simulink model "gm_sampleModel1671_3_sub"  (R2023a)
settings: Solver=VariableStepAuto  StartTime=0.0  StopTime=10.0  RelTol=1e-3
libraries: simulink x1, hdlsllib x1
settings Model: Creator=user1  LastModifiedBy=user1
settings OptimizationCC: BlockReduction=off  ConditionallyExecuteInputs=off
settings DebuggingCC: InheritedTsInSrcMsg=none

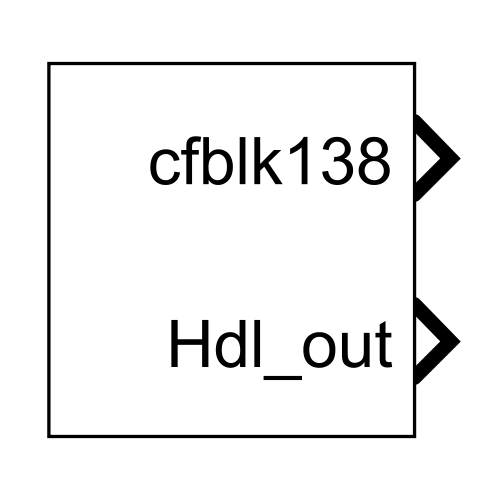
[thumbnail: Simulink's stored preview of the top-level diagram]
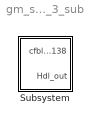
== system gm_sampleModel1671_3_sub ==
  Subsystem : Subsystem

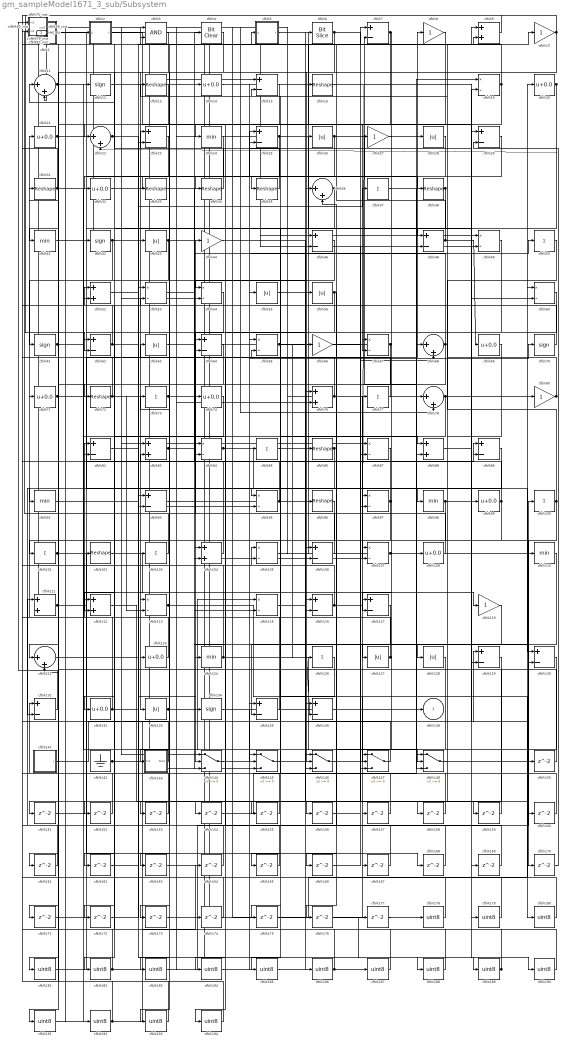
== system gm_sampleModel1671_3_sub/Subsystem ==
  cfblk1 : Subsystem  mask(Detect Fall Negative){vinit=double(0), InputProcessing=Elements as channels (sample based), OutDataTypeStr=uint8}
      mask prompts: vinit "Simulink:masks:InitialCondition_MP"; InputProcessing "Simulink:masks:InputProcessing_MP"; OutDataTypeStr "Simulink:masks:OutputDataType_MP"
      mask help: Simulink:masks:DetectFallNegative_MD
      mask init:
      | InputProcessing = 'Elements as channels (sample based)';
      | OutDataTypeStr = 'uint8';
      | vinit = double(0);
      mask TypeOptions InputProcessing: Simulink:masks:ColumnsAsChannelsFrameBased | Simulink:masks:ElementsAsChannelsSampleBased
      mask TypeOptions OutDataTypeStr: Simulink:masks:uint8 | Simulink:masks:boolean
      mask Display: fprintf('U < 0\n&  NOT\nU/z < 0')
  cfblk{8,10,27,44,66,80,119} (7 alike) : Gain  OutDataTypeStr=uint8
  cfblk{37,50,73,77,85,100..101,103,126} (9 alike) : Sum  Inputs=+  OutDataTypeStr=uint8
  cfblk{13,16,31,33..35,38,72,86,96,102} (11 alike) : Reshape
  cfblk{9,52,76,83,88,104,111..112} (8 alike) : Sum  OutDataTypeStr=uint8
  cfblk{19,49,53..54,60,65,67,84,87,95,97,105,107,113,115} (15 alike) : Product  Inputs=*/  OutDataTypeStr=uint8  RndMeth=Zero  SaturateOnIntegerOverflow=on
  cfblk{7,15,23,25,29,46,48,62,64,82,89,93,106,116..117,129..131,135..136} (20 alike) : Sum  Inputs=+-  OutDataTypeStr=uint8
  cfblk{14,20..21,32,69,71,74,99,108,123,132} (11 alike) : Bias  Bias=0.0  SaturateOnIntegerOverflow=off
  cfblk{11,22,36,68,78,121} (6 alike) : Sum  Inputs=|++  OutDataTypeStr=uint8
  cfblk{24,41,91,98,110,124} (6 alike) : MinMax  OutDataTypeStr=uint8
  cfblk114_inst : Subsystem
  cfblk118_inst : Subsystem
  cfblk{12,42,61,70,134} (5 alike) : Signum
  cfblk122_inst : Subsystem
  cfblk125_inst : Subsystem
  cfblk{26,28,43,55..56,63,127..128,133} (9 alike) : Abs  OutDataTypeStr=uint8  SaturateOnIntegerOverflow=off
  cfblk141 : Subsystem  mask(Counter Limited){uplimit=double(7), tsamp=double(-1)}
      mask prompts: uplimit "Simulink:masks:UpperLimit_MP"; tsamp "Simulink:masks:SampleTime_MP"
      mask help: Simulink:masks:CounterLimited_MD
      mask init:
      | nbits = double(8);
      | tsamp = double(-1);
      | uplimit = double(7);
  cfblk142 : Ground
  cfblk143 : Subsystem
  cfblk{144..148} (5 alike) : Switch  OutDataTypeStr=uint8  SaturateOnIntegerOverflow=off  InputSameDT=off
  cfblk{150..177} (28 alike) : Delay  SampleTime=1
  cfblk{178..194} (17 alike) : DataTypeConversion  OutDataTypeStr=uint8  SaturateOnIntegerOverflow=off  RndMeth=Floor
  cfblk17_inst : Subsystem
  cfblk18_inst : Subsystem
  cfblk2 : Subsystem  mask(Detect Fall Nonpositive){vinit=double(0), InputProcessing=Elements as channels (sample based), OutDataTypeStr=uint8}
      mask prompts: vinit "Simulink:masks:InitialCondition_MP"; InputProcessing "Simulink:masks:InputProcessing_MP"; OutDataTypeStr "Simulink:masks:OutputDataType_MP"
      mask help: Simulink:masks:DetectFallNonpositive_MD
      mask init:
      | InputProcessing = 'Elements as channels (sample based)';
      | OutDataTypeStr = 'uint8';
      | vinit = double(0);
      mask TypeOptions InputProcessing: Simulink:masks:ColumnsAsChannelsFrameBased | Simulink:masks:ElementsAsChannelsSampleBased
      mask TypeOptions OutDataTypeStr: Simulink:masks:uint8 | Simulink:masks:boolean
      mask Display: fprintf('U <= 0\n&  NOT\nU/z <= 0')
  cfblk3 : Logic  AllPortsSameDT=off  OutDataTypeStr=boolean
  cfblk30_inst : Subsystem
  cfblk39_inst : Subsystem
  cfblk4 : simulink/Logic and Bit Operations/Bit Clear  iBit=0
      settings: LibrarySourceBlock=|
      | hdlsllib/Logic and Bit
      | Operations/Bit Clear
  cfblk40_inst : Subsystem
  cfblk45_inst : Subsystem
  cfblk47_inst : Subsystem
  cfblk5 : Subsystem  mask(Detect Fall Negative){vinit=double(0), InputProcessing=Elements as channels (sample based), OutDataTypeStr=uint8}
      mask prompts: vinit "Simulink:masks:InitialCondition_MP"; InputProcessing "Simulink:masks:InputProcessing_MP"; OutDataTypeStr "Simulink:masks:OutputDataType_MP"
      mask help: Simulink:masks:DetectFallNegative_MD
      mask init:
      | InputProcessing = 'Elements as channels (sample based)';
      | OutDataTypeStr = 'uint8';
      | vinit = double(0);
      mask TypeOptions InputProcessing: Simulink:masks:ColumnsAsChannelsFrameBased | Simulink:masks:ElementsAsChannelsSampleBased
      mask TypeOptions OutDataTypeStr: Simulink:masks:uint8 | Simulink:masks:boolean
      mask Display: fprintf('U < 0\n&  NOT\nU/z < 0')
  cfblk51_inst : Subsystem
  cfblk57_inst : Subsystem
  cfblk59_inst : Subsystem
  cfblk6 : hdlsllib/Logic and Bit Operations/Bit Slice  lidx=7  ridx=0
  cfblk75_inst : Subsystem
  cfblk79_inst : Subsystem
  cfblk90_inst : Subsystem
  cfblk92_inst : Subsystem
  cfblk138 : Outport  OutDataTypeStr=uint8  SampleTime=1  VectorParamsAs1DForOutWhenUnconnected=off
  Hdl_out : Outport  Port=2  OutDataTypeStr=uint8  SampleTime=1
  wires:
  cfblk1/1(Y) -> cfblk88/1, cfblk95/1
  cfblk10/1 -> cfblk62/2, cfblk146/2, cfblk133/1
  cfblk100/1 -> cfblk123/1, cfblk53/2, cfblk170/1
  cfblk101/1 -> cfblk8/1, cfblk168/1
  cfblk102/1 -> cfblk116/1
  cfblk103/1 -> cfblk59_inst/2(in2)
  cfblk104/1 -> cfblk83/2
  cfblk105/1 -> cfblk10/1
  cfblk106/1 -> cfblk44/1
  cfblk107/1 -> cfblk108/1, cfblk19/1
  cfblk108/1 -> cfblk23/1
  cfblk11/1 -> cfblk76/1, cfblk144/2
  cfblk110/1 -> cfblk135/2
  cfblk111/1 -> cfblk12/1, cfblk65/2
  cfblk112/1 -> cfblk154/1
  cfblk113/1 -> cfblk55/1, cfblk180/1
  cfblk114_inst/1(out1) -> cfblk186/1
  cfblk115/1 -> cfblk106/2
  cfblk116/1 -> cfblk7/2, cfblk45_inst/2(in2)
  cfblk117/1 -> cfblk185/1
  cfblk118_inst/1(out1) -> cfblk192/1
  cfblk119/1 -> cfblk128/1
  cfblk12/1 -> cfblk24/1
  cfblk121/1 -> cfblk146/1
  cfblk122_inst/1(out1) -> cfblk84/1
  cfblk123/1 -> cfblk21/1
  cfblk124/1 -> cfblk71/1, cfblk148/2, cfblk136/2, cfblk177/1
  cfblk125_inst/1(out1) -> cfblk74/1, cfblk111/2, cfblk11/2
  cfblk126/1 -> cfblk165/1
  cfblk127/1 -> cfblk82/1, cfblk15/2
  cfblk128/1 -> cfblk166/1
  cfblk129/1 -> cfblk151/1
  cfblk13/1 -> cfblk41/1
  cfblk130/1 -> cfblk167/1
  cfblk131/1 -> cfblk79_inst/1(in1)
  cfblk132/1 -> cfblk40_inst/2(in2), cfblk159/1
  cfblk133/1 -> cfblk146/3, cfblk115/1
  cfblk134/1 -> cfblk145/1
  cfblk135/1 -> cfblk57_inst/1(in1)
  cfblk136/1 -> cfblk78/1
  cfblk14/1 -> cfblk38/1
  cfblk141/1(y) -> cfblk116/2
  cfblk142/1 -> cfblk129/1, cfblk19/2
  cfblk143/1(Out1) -> cfblk125_inst/1(in1)
  cfblk144/1 -> cfblk70/1
  cfblk145/1 -> cfblk157/1
  cfblk146/1 -> cfblk77/1
  cfblk147/1 -> cfblk136/1
  cfblk148/1 -> cfblk100/1
  cfblk15/1 -> cfblk54/1
  cfblk150/1 -> cfblk122_inst/2(in2)
  cfblk151/1 -> cfblk25/2
  cfblk152/1 -> cfblk131/1
  cfblk153/1 -> cfblk79_inst/2(in2)
  cfblk154/1 -> cfblk88/2
  cfblk155/1 -> cfblk84/2
  cfblk156/1 -> cfblk68/1
  cfblk157/1 -> cfblk57_inst/2(in2)
  cfblk158/1 -> cfblk51_inst/1(in1)
  cfblk159/1 -> cfblk75_inst/1(in1)
  cfblk16/1 -> cfblk190/1
  cfblk160/1 -> cfblk105/1
  cfblk161/1 -> cfblk40_inst/1(in1)
  cfblk162/1 -> cfblk93/1
  cfblk163/1 -> cfblk135/1
  cfblk164/1 -> cfblk3/1
  cfblk165/1 -> cfblk92_inst/2(in2)
  cfblk166/1 -> cfblk48/2
  cfblk167/1 -> cfblk64/1
  cfblk168/1 -> cfblk111/1
  cfblk169/1 -> cfblk36/2
  cfblk17_inst/1(out1) -> cfblk43/1, cfblk138/1
  cfblk170/1 -> cfblk29/2
  cfblk171/1 -> cfblk23/2
  cfblk172/1 -> cfblk83/1
  cfblk173/1 -> cfblk46/2
  cfblk174/1 -> cfblk62/1
  cfblk175/1 -> cfblk60/1
  cfblk176/1 -> cfblk188/1
  cfblk177/1 -> cfblk1/1(U)
  cfblk178/1 -> cfblk53/1
  cfblk179/1 -> cfblk18_inst/1(in1)
  cfblk18_inst/1(out1) -> cfblk178/1
  cfblk180/1 -> cfblk18_inst/2(in2)
  cfblk181/1 -> cfblk4/1
  cfblk182/1 -> cfblk17_inst/2(in2), cfblk105/2
  cfblk183/1 -> cfblk150/1
  cfblk184/1 -> cfblk89/1
  cfblk185/1 -> cfblk89/2
  cfblk186/1 -> cfblk39_inst/2(in2), cfblk122_inst/1(in1)
  cfblk187/1 -> cfblk114_inst/1(in1)
  cfblk188/1 -> cfblk114_inst/2(in2)
  cfblk189/1 -> cfblk90_inst/2(in2), cfblk164/1
  cfblk19/1 -> cfblk45_inst/1(in1), cfblk147/2
  cfblk190/1 -> cfblk52/1
  cfblk191/1 -> cfblk52/2
  cfblk192/1 -> cfblk31/1, cfblk20/1, cfblk174/1
  cfblk193/1 -> cfblk118_inst/1(in1)
  cfblk194/1 -> cfblk118_inst/2(in2)
  cfblk2/1(Y) -> cfblk179/1
  cfblk20/1 -> cfblk22/2, cfblk144/3, cfblk175/1
  cfblk21/1 -> cfblk48/1, cfblk34/1
  cfblk22/1 -> cfblk147/3, cfblk134/1
  cfblk23/1 -> cfblk72/1
  cfblk24/1 -> cfblk193/1
  cfblk25/1 -> cfblk99/1, cfblk93/2
  cfblk26/1 -> cfblk9/2, cfblk148/1, cfblk173/1, cfblk172/1
  cfblk27/1 -> cfblk107/1
  cfblk28/1 -> cfblk36/1
  cfblk29/1 -> cfblk32/1
  cfblk3/1 -> cfblk191/1
  cfblk30_inst/1(out1) -> cfblk42/1
  cfblk31/1 -> cfblk39_inst/1(in1), cfblk171/1, cfblk113/1
  cfblk32/1 -> cfblk35/1
  cfblk33/1 -> cfblk56/1
  cfblk34/1 -> cfblk11/1
  cfblk35/1 -> cfblk51_inst/2(in2)
  cfblk36/1 -> cfblk194/1, cfblk124/1
  cfblk37/1 -> cfblk129/2
  cfblk38/1 -> cfblk112/2, cfblk153/1
  cfblk39_inst/1(out1) -> cfblk26/1, cfblk144/1
  cfblk4/1 -> cfblk182/1
  cfblk40_inst/1(out1) -> cfblk76/2, cfblk54/2
  cfblk41/1 -> cfblk102/1
  cfblk42/1 -> cfblk121/2, cfblk5/1(U)
  cfblk43/1 -> cfblk7/1, cfblk61/1
  cfblk44/1 -> cfblk147/1
  cfblk45_inst/1(out1) -> cfblk14/1
  cfblk46/1 -> cfblk132/1
  cfblk47_inst/1(out1) -> cfblk95/2, cfblk2/1(U)
  cfblk48/1 -> cfblk69/1, cfblk47_inst/1(in1)
  cfblk49/1 -> cfblk97/1
  cfblk5/1(Y) -> cfblk67/2
  cfblk50/1 -> cfblk158/1
  cfblk51_inst/1(out1) -> cfblk187/1, cfblk27/1
  cfblk52/1 -> cfblk189/1
  cfblk53/1 -> cfblk97/2
  cfblk54/1 -> cfblk64/2
  cfblk55/1 -> cfblk6/1
  cfblk56/1 -> cfblk104/1, cfblk176/1
  cfblk57_inst/1(out1) -> cfblk28/1, cfblk87/1
  cfblk59_inst/1(out1) -> cfblk30_inst/1(in1), cfblk145/3
  cfblk6/1 -> cfblk148/3, cfblk163/1
  cfblk60/1 -> cfblk66/1
  cfblk61/1 -> cfblk117/2, cfblk161/1
  cfblk62/1 -> cfblk33/1, cfblk30_inst/2(in2)
  cfblk63/1 -> cfblk50/1
  cfblk64/1 -> cfblk143/1(In1)
  cfblk65/1 -> cfblk130/2, cfblk119/1, cfblk126/1
  cfblk66/1 -> cfblk68/2
  cfblk67/1 -> cfblk121/1, cfblk117/1, Hdl_out/1
  cfblk68/1 -> cfblk25/1, cfblk112/1
  cfblk69/1 -> cfblk98/1
  cfblk7/1 -> cfblk67/1, cfblk103/1
  cfblk70/1 -> cfblk90_inst/1(in1)
  cfblk71/1 -> cfblk145/2, cfblk87/2
  cfblk72/1 -> cfblk92_inst/1(in1), cfblk113/2
  cfblk73/1 -> cfblk9/1, cfblk3/2, cfblk115/2
  cfblk74/1 -> cfblk162/1
  cfblk75_inst/1(out1) -> cfblk80/1, cfblk49/1, cfblk107/2
  cfblk76/1 -> cfblk17_inst/1(in1), cfblk160/1
  cfblk77/1 -> cfblk63/1
  cfblk78/1 -> cfblk156/1, cfblk155/1
  cfblk79_inst/1(out1) -> cfblk75_inst/2(in2), cfblk16/1, cfblk49/2
  cfblk8/1 -> cfblk22/1
  cfblk80/1 -> cfblk47_inst/2(in2), cfblk13/1
  cfblk82/1 -> cfblk65/1
  cfblk83/1 -> cfblk46/1, cfblk127/1
  cfblk84/1 -> cfblk130/1, cfblk85/1
  cfblk85/1 -> cfblk86/1
  cfblk86/1 -> cfblk184/1, cfblk131/2
  cfblk87/1 -> cfblk181/1
  cfblk88/1 -> cfblk60/2
  cfblk89/1 -> cfblk183/1
  cfblk9/1 -> cfblk59_inst/1(in1)
  cfblk90_inst/1(out1) -> cfblk96/1
  cfblk91/1 -> cfblk37/1
  cfblk92_inst/1(out1) -> cfblk78/2, cfblk15/1, cfblk110/1
  cfblk93/1 -> cfblk29/1
  cfblk95/1 -> cfblk82/2, cfblk73/1
  cfblk96/1 -> cfblk106/1
  cfblk97/1 -> cfblk152/1, cfblk91/1
  cfblk98/1 -> cfblk169/1, cfblk101/1
  cfblk99/1 -> cfblk125_inst/2(in2), cfblk104/2

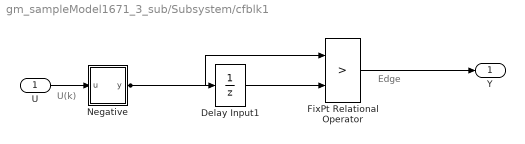
== system gm_sampleModel1671_3_sub/Subsystem/cfblk1 ==
  note: U(k)
  note: Edge
  U : Inport  OutDataTypeStr=uint8  SampleTime=1
  Delay Input1 : UnitDelay  Description=Store in Global RAM  DisableCoverage=on  InitialCondition=vinit  SampleTime=-1  HasFrameUpgradeWarning=on
  FixPt Relational Operator : RelationalOperator  Operator=>  OutDataTypeStr=fixdt(0, 8)  ZeroCross=off  InputSameDT=off
  Negative : Subsystem  mask(Compare To Zero){relop=<, OutDataTypeStr=boolean, ZeroCross=off}
      mask prompts: relop "Simulink:masks:Operator_MP"; OutDataTypeStr "Simulink:masks:OutputDataType_MP"; ZeroCross "Simulink:masks:EnableZerocrossingDetection_MP"
      mask help: Simulink:masks:CompareToZero_MD
      mask init:
      | OutDataTypeStr = 'boolean';
      | ZeroCross = 'off';
      | blkName = 'sampleModel1671_3_sub/Subsystem/cfblk1/Negative';
      | relop = '<';
      | setValue = 'boolean';
      mask TypeOptions relop: == | ~= | < | <= | >= | >
      mask TypeOptions OutDataTypeStr: Simulink:masks:uint8 | Simulink:masks:boolean
      mask Callback ZeroCross: sl('zeroCrossEnable', gcbh);
      mask Display: disp([relop,' 0'])
  Y : Outport  SampleTime=1
  wires:
  U/1 -> Negative/1(u)
  Delay Input1/1 -> FixPt Relational Operator/2
  FixPt Relational Operator/1 -> Y/1
  Negative/1(y) -> FixPt Relational Operator/1, Delay Input1/1

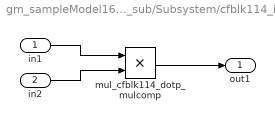
== system gm_sampleModel1671_3_sub/Subsystem/cfblk114_inst ==
  in1 : Inport  OutDataTypeStr=uint8  SampleTime=1
  in2 : Inport  Port=2  OutDataTypeStr=uint8  SampleTime=1
  mul_cfblk114_dotp_mulcomp : Product  Inputs=**  OutDataTypeStr=uint8  SampleTime=1
  out1 : Outport  OutDataTypeStr=uint8  SampleTime=1
  wires:
  in1/1 -> mul_cfblk114_dotp_mulcomp/1
  in2/1 -> mul_cfblk114_dotp_mulcomp/2
  mul_cfblk114_dotp_mulcomp/1 -> out1/1

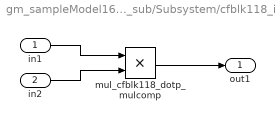
== system gm_sampleModel1671_3_sub/Subsystem/cfblk118_inst ==
  in1 : Inport  OutDataTypeStr=uint8  SampleTime=1
  in2 : Inport  Port=2  OutDataTypeStr=uint8  SampleTime=1
  mul_cfblk118_dotp_mulcomp : Product  Inputs=**  OutDataTypeStr=uint8  SampleTime=1
  out1 : Outport  OutDataTypeStr=uint8  SampleTime=1
  wires:
  in1/1 -> mul_cfblk118_dotp_mulcomp/1
  in2/1 -> mul_cfblk118_dotp_mulcomp/2
  mul_cfblk118_dotp_mulcomp/1 -> out1/1

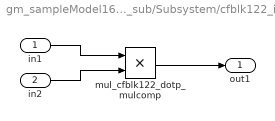
== system gm_sampleModel1671_3_sub/Subsystem/cfblk122_inst ==
  in1 : Inport  OutDataTypeStr=uint8  SampleTime=1
  in2 : Inport  Port=2  OutDataTypeStr=uint8  SampleTime=1
  mul_cfblk122_dotp_mulcomp : Product  Inputs=**  OutDataTypeStr=uint8  SampleTime=1
  out1 : Outport  OutDataTypeStr=uint8  SampleTime=1
  wires:
  in1/1 -> mul_cfblk122_dotp_mulcomp/1
  in2/1 -> mul_cfblk122_dotp_mulcomp/2
  mul_cfblk122_dotp_mulcomp/1 -> out1/1

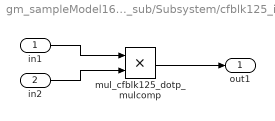
== system gm_sampleModel1671_3_sub/Subsystem/cfblk125_inst ==
  in1 : Inport  OutDataTypeStr=uint8  SampleTime=1
  in2 : Inport  Port=2  OutDataTypeStr=uint8  SampleTime=1
  mul_cfblk125_dotp_mulcomp : Product  Inputs=**  OutDataTypeStr=uint8  SampleTime=1
  out1 : Outport  OutDataTypeStr=uint8  SampleTime=1
  wires:
  in1/1 -> mul_cfblk125_dotp_mulcomp/1
  in2/1 -> mul_cfblk125_dotp_mulcomp/2
  mul_cfblk125_dotp_mulcomp/1 -> out1/1

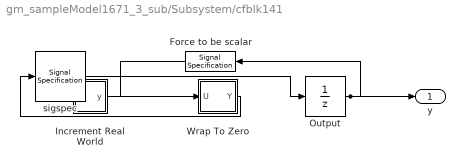
== system gm_sampleModel1671_3_sub/Subsystem/cfblk141 ==
  Force to be scalar : SignalSpecification  DisableCoverage=on  Dimensions=1
  Increment Real World : Subsystem  mask(Real World Value Increment){}
      mask help: Simulink:masks:RealWorldValueIncrement_MD
      mask Display: disp('V++')
  Output : UnitDelay  InitialCondition=0.0  SampleTime=tsamp  HasFrameUpgradeWarning=on
  Wrap To Zero : Subsystem  mask(Wrap To Zero){Threshold=double(7)}
      mask prompts: Threshold "Simulink:masks:Threshold_MP"
      mask help: Simulink:masks:WrapToZero_MD
  sigspec : SignalSpecification  OutDataTypeStr=uint8  Dimensions=1
  y : Outport  SampleTime=1
  wires:
  Force to be scalar/1 -> Increment Real World/1(u)
  Increment Real World/1(y) -> Wrap To Zero/1(U)
  Output/1 -> Force to be scalar/1, y/1
  Wrap To Zero/1(Y) -> sigspec/1
  sigspec/1 -> Output/1

== system gm_sampleModel1671_3_sub/Subsystem/cfblk143 ==
  In1 : Inport  OutDataTypeStr=uint8  PortDimensions=1  SampleTime=1
  Out1 : Outport  SampleTime=1
  wires:
  In1/1 -> Out1/1

== system gm_sampleModel1671_3_sub/Subsystem/cfblk17_inst ==
  in1 : Inport  OutDataTypeStr=uint8  SampleTime=1
  in2 : Inport  Port=2  OutDataTypeStr=uint8  SampleTime=1
  mul_cfblk17_dotp_mulcomp : Product  Inputs=**  OutDataTypeStr=uint8  SampleTime=1
  out1 : Outport  OutDataTypeStr=uint8  SampleTime=1
  wires:
  in1/1 -> mul_cfblk17_dotp_mulcomp/1
  in2/1 -> mul_cfblk17_dotp_mulcomp/2
  mul_cfblk17_dotp_mulcomp/1 -> out1/1

== system gm_sampleModel1671_3_sub/Subsystem/cfblk18_inst ==
  in1 : Inport  OutDataTypeStr=uint8  SampleTime=1
  in2 : Inport  Port=2  OutDataTypeStr=uint8  SampleTime=1
  mul_cfblk18_dotp_mulcomp : Product  Inputs=**  OutDataTypeStr=uint8  SampleTime=1
  out1 : Outport  OutDataTypeStr=uint8  SampleTime=1
  wires:
  in1/1 -> mul_cfblk18_dotp_mulcomp/1
  in2/1 -> mul_cfblk18_dotp_mulcomp/2
  mul_cfblk18_dotp_mulcomp/1 -> out1/1

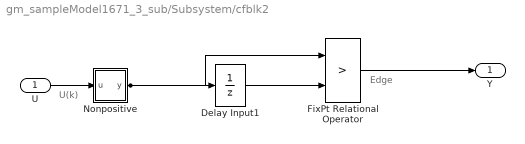
== system gm_sampleModel1671_3_sub/Subsystem/cfblk2 ==
  note: U(k)
  note: Edge
  U : Inport  OutDataTypeStr=uint8  SampleTime=1
  Delay Input1 : UnitDelay  Description=Store in Global RAM  DisableCoverage=on  InitialCondition=vinit  SampleTime=-1  HasFrameUpgradeWarning=on
  FixPt Relational Operator : RelationalOperator  Operator=>  OutDataTypeStr=fixdt(0, 8)  ZeroCross=off  InputSameDT=off
  Nonpositive : Subsystem  mask(Compare To Zero){relop=<=, OutDataTypeStr=boolean, ZeroCross=off}
      mask prompts: relop "Simulink:masks:Operator_MP"; OutDataTypeStr "Simulink:masks:OutputDataType_MP"; ZeroCross "Simulink:masks:EnableZerocrossingDetection_MP"
      mask help: Simulink:masks:CompareToZero_MD
      mask init:
      | OutDataTypeStr = 'boolean';
      | ZeroCross = 'off';
      | blkName = 'sampleModel1671_3_sub/Subsystem/cfblk2/Nonpositive';
      | relop = '<=';
      | setValue = 'boolean';
      mask TypeOptions relop: == | ~= | < | <= | >= | >
      mask TypeOptions OutDataTypeStr: Simulink:masks:uint8 | Simulink:masks:boolean
      mask Callback ZeroCross: sl('zeroCrossEnable', gcbh);
      mask Display: disp([relop,' 0'])
  Y : Outport  SampleTime=1
  wires:
  U/1 -> Nonpositive/1(u)
  Delay Input1/1 -> FixPt Relational Operator/2
  FixPt Relational Operator/1 -> Y/1
  Nonpositive/1(y) -> FixPt Relational Operator/1, Delay Input1/1

== system gm_sampleModel1671_3_sub/Subsystem/cfblk30_inst ==
  in1 : Inport  OutDataTypeStr=uint8  SampleTime=1
  in2 : Inport  Port=2  OutDataTypeStr=uint8  SampleTime=1
  mul_cfblk30_dotp_mulcomp : Product  Inputs=**  OutDataTypeStr=uint8  SampleTime=1
  out1 : Outport  OutDataTypeStr=uint8  SampleTime=1
  wires:
  in1/1 -> mul_cfblk30_dotp_mulcomp/1
  in2/1 -> mul_cfblk30_dotp_mulcomp/2
  mul_cfblk30_dotp_mulcomp/1 -> out1/1

== system gm_sampleModel1671_3_sub/Subsystem/cfblk39_inst ==
  in1 : Inport  OutDataTypeStr=uint8  SampleTime=1
  in2 : Inport  Port=2  OutDataTypeStr=uint8  SampleTime=1
  mul_cfblk39_dotp_mulcomp : Product  Inputs=**  OutDataTypeStr=uint8  SampleTime=1
  out1 : Outport  OutDataTypeStr=uint8  SampleTime=1
  wires:
  in1/1 -> mul_cfblk39_dotp_mulcomp/1
  in2/1 -> mul_cfblk39_dotp_mulcomp/2
  mul_cfblk39_dotp_mulcomp/1 -> out1/1

== system gm_sampleModel1671_3_sub/Subsystem/cfblk40_inst ==
  in1 : Inport  OutDataTypeStr=uint8  SampleTime=1
  in2 : Inport  Port=2  OutDataTypeStr=uint8  SampleTime=1
  mul_cfblk40_dotp_mulcomp : Product  Inputs=**  OutDataTypeStr=uint8  SampleTime=1
  out1 : Outport  OutDataTypeStr=uint8  SampleTime=1
  wires:
  in1/1 -> mul_cfblk40_dotp_mulcomp/1
  in2/1 -> mul_cfblk40_dotp_mulcomp/2
  mul_cfblk40_dotp_mulcomp/1 -> out1/1

== system gm_sampleModel1671_3_sub/Subsystem/cfblk45_inst ==
  in1 : Inport  OutDataTypeStr=uint8  SampleTime=1
  in2 : Inport  Port=2  OutDataTypeStr=uint8  SampleTime=1
  mul_cfblk45_dotp_mulcomp : Product  Inputs=**  OutDataTypeStr=uint8  SampleTime=1
  out1 : Outport  OutDataTypeStr=uint8  SampleTime=1
  wires:
  in1/1 -> mul_cfblk45_dotp_mulcomp/1
  in2/1 -> mul_cfblk45_dotp_mulcomp/2
  mul_cfblk45_dotp_mulcomp/1 -> out1/1

== system gm_sampleModel1671_3_sub/Subsystem/cfblk47_inst ==
  in1 : Inport  OutDataTypeStr=uint8  SampleTime=1
  in2 : Inport  Port=2  OutDataTypeStr=uint8  SampleTime=1
  mul_cfblk47_dotp_mulcomp : Product  Inputs=**  OutDataTypeStr=uint8  SampleTime=1
  out1 : Outport  OutDataTypeStr=uint8  SampleTime=1
  wires:
  in1/1 -> mul_cfblk47_dotp_mulcomp/1
  in2/1 -> mul_cfblk47_dotp_mulcomp/2
  mul_cfblk47_dotp_mulcomp/1 -> out1/1

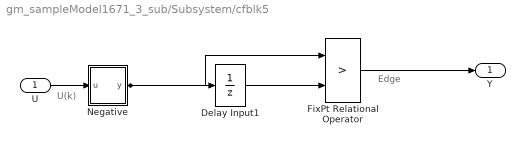
== system gm_sampleModel1671_3_sub/Subsystem/cfblk5 ==
  note: U(k)
  note: Edge
  U : Inport  OutDataTypeStr=uint8  SampleTime=1
  Delay Input1 : UnitDelay  Description=Store in Global RAM  DisableCoverage=on  InitialCondition=vinit  SampleTime=-1  HasFrameUpgradeWarning=on
  FixPt Relational Operator : RelationalOperator  Operator=>  OutDataTypeStr=fixdt(0, 8)  ZeroCross=off  InputSameDT=off
  Negative : Subsystem  mask(Compare To Zero){relop=<, OutDataTypeStr=boolean, ZeroCross=off}
      mask prompts: relop "Simulink:masks:Operator_MP"; OutDataTypeStr "Simulink:masks:OutputDataType_MP"; ZeroCross "Simulink:masks:EnableZerocrossingDetection_MP"
      mask help: Simulink:masks:CompareToZero_MD
      mask init:
      | OutDataTypeStr = 'boolean';
      | ZeroCross = 'off';
      | blkName = 'sampleModel1671_3_sub/Subsystem/cfblk5/Negative';
      | relop = '<';
      | setValue = 'boolean';
      mask TypeOptions relop: == | ~= | < | <= | >= | >
      mask TypeOptions OutDataTypeStr: Simulink:masks:uint8 | Simulink:masks:boolean
      mask Callback ZeroCross: sl('zeroCrossEnable', gcbh);
      mask Display: disp([relop,' 0'])
  Y : Outport  SampleTime=1
  wires:
  U/1 -> Negative/1(u)
  Delay Input1/1 -> FixPt Relational Operator/2
  FixPt Relational Operator/1 -> Y/1
  Negative/1(y) -> FixPt Relational Operator/1, Delay Input1/1

== system gm_sampleModel1671_3_sub/Subsystem/cfblk51_inst ==
  in1 : Inport  OutDataTypeStr=uint8  SampleTime=1
  in2 : Inport  Port=2  OutDataTypeStr=uint8  SampleTime=1
  mul_cfblk51_dotp_mulcomp : Product  Inputs=**  OutDataTypeStr=uint8  SampleTime=1
  out1 : Outport  OutDataTypeStr=uint8  SampleTime=1
  wires:
  in1/1 -> mul_cfblk51_dotp_mulcomp/1
  in2/1 -> mul_cfblk51_dotp_mulcomp/2
  mul_cfblk51_dotp_mulcomp/1 -> out1/1

== system gm_sampleModel1671_3_sub/Subsystem/cfblk57_inst ==
  in1 : Inport  OutDataTypeStr=uint8  SampleTime=1
  in2 : Inport  Port=2  OutDataTypeStr=uint8  SampleTime=1
  mul_cfblk57_dotp_mulcomp : Product  Inputs=**  OutDataTypeStr=uint8  SampleTime=1
  out1 : Outport  OutDataTypeStr=uint8  SampleTime=1
  wires:
  in1/1 -> mul_cfblk57_dotp_mulcomp/1
  in2/1 -> mul_cfblk57_dotp_mulcomp/2
  mul_cfblk57_dotp_mulcomp/1 -> out1/1

== system gm_sampleModel1671_3_sub/Subsystem/cfblk59_inst ==
  in1 : Inport  OutDataTypeStr=uint8  SampleTime=1
  in2 : Inport  Port=2  OutDataTypeStr=uint8  SampleTime=1
  mul_cfblk59_dotp_mulcomp : Product  Inputs=**  OutDataTypeStr=uint8  SampleTime=1
  out1 : Outport  OutDataTypeStr=uint8  SampleTime=1
  wires:
  in1/1 -> mul_cfblk59_dotp_mulcomp/1
  in2/1 -> mul_cfblk59_dotp_mulcomp/2
  mul_cfblk59_dotp_mulcomp/1 -> out1/1

== system gm_sampleModel1671_3_sub/Subsystem/cfblk75_inst ==
  in1 : Inport  OutDataTypeStr=uint8  SampleTime=1
  in2 : Inport  Port=2  OutDataTypeStr=uint8  SampleTime=1
  mul_cfblk75_dotp_mulcomp : Product  Inputs=**  OutDataTypeStr=uint8  SampleTime=1
  out1 : Outport  OutDataTypeStr=uint8  SampleTime=1
  wires:
  in1/1 -> mul_cfblk75_dotp_mulcomp/1
  in2/1 -> mul_cfblk75_dotp_mulcomp/2
  mul_cfblk75_dotp_mulcomp/1 -> out1/1

== system gm_sampleModel1671_3_sub/Subsystem/cfblk79_inst ==
  in1 : Inport  OutDataTypeStr=uint8  SampleTime=1
  in2 : Inport  Port=2  OutDataTypeStr=uint8  SampleTime=1
  mul_cfblk79_dotp_mulcomp : Product  Inputs=**  OutDataTypeStr=uint8  SampleTime=1
  out1 : Outport  OutDataTypeStr=uint8  SampleTime=1
  wires:
  in1/1 -> mul_cfblk79_dotp_mulcomp/1
  in2/1 -> mul_cfblk79_dotp_mulcomp/2
  mul_cfblk79_dotp_mulcomp/1 -> out1/1

== system gm_sampleModel1671_3_sub/Subsystem/cfblk90_inst ==
  in1 : Inport  OutDataTypeStr=uint8  SampleTime=1
  in2 : Inport  Port=2  OutDataTypeStr=uint8  SampleTime=1
  mul_cfblk90_dotp_mulcomp : Product  Inputs=**  OutDataTypeStr=uint8  SampleTime=1
  out1 : Outport  OutDataTypeStr=uint8  SampleTime=1
  wires:
  in1/1 -> mul_cfblk90_dotp_mulcomp/1
  in2/1 -> mul_cfblk90_dotp_mulcomp/2
  mul_cfblk90_dotp_mulcomp/1 -> out1/1

== system gm_sampleModel1671_3_sub/Subsystem/cfblk92_inst ==
  in1 : Inport  OutDataTypeStr=uint8  SampleTime=1
  in2 : Inport  Port=2  OutDataTypeStr=uint8  SampleTime=1
  mul_cfblk92_dotp_mulcomp : Product  Inputs=**  OutDataTypeStr=uint8  SampleTime=1
  out1 : Outport  OutDataTypeStr=uint8  SampleTime=1
  wires:
  in1/1 -> mul_cfblk92_dotp_mulcomp/1
  in2/1 -> mul_cfblk92_dotp_mulcomp/2
  mul_cfblk92_dotp_mulcomp/1 -> out1/1

== system gm_sampleModel1671_3_sub/Subsystem/cfblk1/Negative ==
  u : Inport  OutDataTypeStr=uint8  SampleTime=1
  Compare : RelationalOperator  Operator=<  OutDataTypeStr=boolean  ZeroCross=off
  Constant : Constant  DisableCoverage=on  Value=0  OutDataTypeStr=Inherit: Inherit via back propagation  SampleTime=-1  PreserveConstantTs=on
  y : Outport  SampleTime=1
  wires:
  u/1 -> Compare/1
  Compare/1 -> y/1
  Constant/1 -> Compare/2

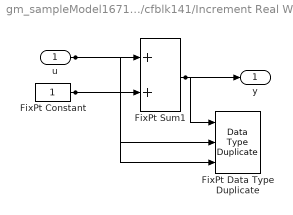
== system gm_sampleModel1671_3_sub/Subsystem/cfblk141/Increment Real World ==
  u : Inport  OutDataTypeStr=uint8  SampleTime=1
  FixPt Constant : Constant  DisableCoverage=on  OutDataTypeStr=Inherit: Inherit via back propagation  SampleTime=-1
  FixPt Data Type Duplicate : DataTypeDuplicate  DisableCoverage=on  NumInputPorts=3
  FixPt Sum1 : Sum  InputSameDT=on  OutDataTypeStr=Inherit: Inherit via back propagation  LockScale=on
  y : Outport  SampleTime=1
  wires:
  u/1 -> FixPt Sum1/1, FixPt Data Type Duplicate/2
  FixPt Constant/1 -> FixPt Sum1/2, FixPt Data Type Duplicate/3
  FixPt Sum1/1 -> FixPt Data Type Duplicate/1, y/1

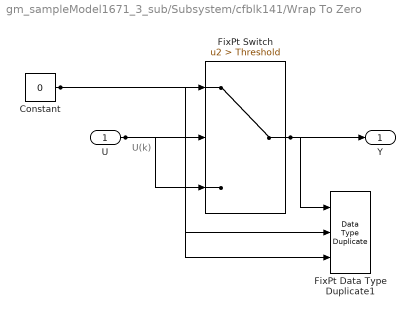
== system gm_sampleModel1671_3_sub/Subsystem/cfblk141/Wrap To Zero ==
  note: U(k)
  U : Inport  OutDataTypeStr=uint8  SampleTime=1
  Constant : Constant  DisableCoverage=on  Value=0  OutDataTypeStr=Inherit: Inherit via back propagation  SampleTime=-1
  FixPt Data Type Duplicate1 : DataTypeDuplicate  DisableCoverage=on  NumInputPorts=3
  FixPt Switch : Switch  Criteria=u2 > Threshold  Threshold=Threshold  OutDataTypeStr=Inherit: Inherit via back propagation  ZeroCross=off  SaturateOnIntegerOverflow=off  InputSameDT=off
  Y : Outport  SampleTime=1
  wires:
  U/1 -> FixPt Switch/3, FixPt Switch/2, FixPt Data Type Duplicate1/2
  Constant/1 -> FixPt Switch/1, FixPt Data Type Duplicate1/3
  FixPt Switch/1 -> FixPt Data Type Duplicate1/1, Y/1

== system gm_sampleModel1671_3_sub/Subsystem/cfblk2/Nonpositive ==
  u : Inport  OutDataTypeStr=uint8  SampleTime=1
  Compare : RelationalOperator  Operator=<=  OutDataTypeStr=boolean  ZeroCross=off
  Constant : Constant  DisableCoverage=on  Value=0  OutDataTypeStr=Inherit: Inherit via back propagation  SampleTime=-1  PreserveConstantTs=on
  y : Outport  SampleTime=1
  wires:
  u/1 -> Compare/1
  Compare/1 -> y/1
  Constant/1 -> Compare/2

== system gm_sampleModel1671_3_sub/Subsystem/cfblk5/Negative ==
  u : Inport  OutDataTypeStr=uint8  SampleTime=1
  Compare : RelationalOperator  Operator=<  OutDataTypeStr=boolean  ZeroCross=off
  Constant : Constant  DisableCoverage=on  Value=0  OutDataTypeStr=Inherit: Inherit via back propagation  SampleTime=-1  PreserveConstantTs=on
  y : Outport  SampleTime=1
  wires:
  u/1 -> Compare/1
  Compare/1 -> y/1
  Constant/1 -> Compare/2
